simulink model "suspension_travel"  (R2021a)
settings: Solver=VariableStepAuto  StartTime=0.0  StopTime=10.0  RelTol=1e-3
settings Model: Creator=admin  LastModifiedBy=admin

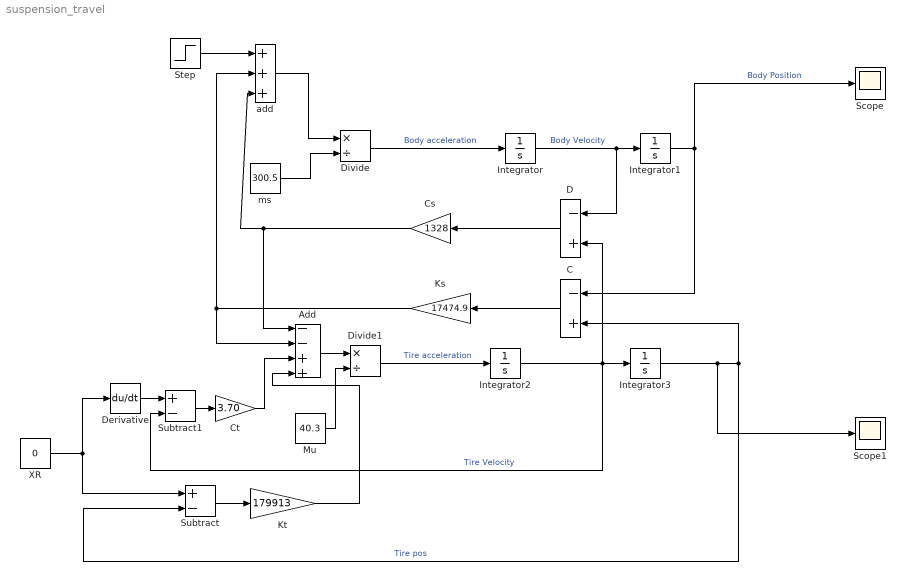
== system suspension_travel ==
  Add : Sum  Inputs=--++
  C : Sum  Inputs=-+
  Cs : Gain  Gain=1328
  Ct : Gain  Gain=3.70
  D : Sum  Inputs=-+
  Derivative : Derivative
  Divide : Product  Inputs=*/
  Divide1 : Product  Inputs=*/
  Integrator{,1..3} (4 alike) : Integrator
  Ks : Gain  Gain=17474.9
  Kt : Gain  Gain=179913
  Mu : Constant  Value=40.3
  Scope : Scope
  Scope1 : Scope
  Step : Step  SampleTime=0
  Subtract : Sum  Inputs=+-
  Subtract1 : Sum  Inputs=+-
  XR : Constant  Value=0
  add : Sum  Inputs=+++
  ms : Constant  Value=300.5
  wires:
  ms/1 -> Divide/2
  Divide/1 -> Integrator/1  "Body acceleration"
  Integrator/1 -> D/1, Integrator1/1  "Body Velocity"
  Cs/1 -> Add/1, add/3
  D/1 -> Cs/1
  Ks/1 -> Add/2, add/2
  C/1 -> Ks/1
  Integrator1/1 -> Scope/1, C/1  "Body Position"
  Mu/1 -> Divide1/2
  Divide1/1 -> Integrator2/1  "Tire acceleration"
  Integrator2/1 -> D/2, Subtract1/2, Integrator3/1  "Tire Velocity"
  XR/1 -> Subtract/1, Derivative/1
  Integrator3/1 -> Scope1/1, C/2, Subtract/2  "Tire pos"
  Subtract/1 -> Kt/1
  Derivative/1 -> Subtract1/1
  Subtract1/1 -> Ct/1
  Ct/1 -> Add/3
  Kt/1 -> Add/4
  Add/1 -> Divide1/1
  Step/1 -> add/1
  add/1 -> Divide/1
